simulink model "SmallScaleMicroGrid"  (R2023b)
settings: Solver=ode23tb  StartTime=0.0  StopTime=24*60*60  FixedStep=1/(1000)  MaxStep=60  RelTol=1e-4
PreLoadFcn:
  | load('SmallScaleMicroGridSolarLoadData24h.mat')
undefined symbols (not defined in the file): Angle, HPD_1min, HPT_1min, Magnitude, SPD_1min, SPT_1min
libraries: spsCurrentMeasurementLib x7, spsControlledCurrentSourceLib x5, spsSeriesRLCBranchLib x5, simulink x4, spsSeriesRLCLoadLib x3, spsVoltageMeasurementLib x2, spsThreePhaseTransformerTwoWindingsLib x1, spsGroundLib x1, spsLinearTransformerLib x1, spsPowerPhasorLib x1, spsThreePhasePISectionLineLib x1, spsThreePhaseSourceLib x1
settings Model: ModifiedByFormat=SPS  Creator=The MathWorks, Inc.  LastModifiedBy=SPS
settings SolverCC: InitialStep=1e-4  ZeroCrossAlgorithm=Adaptive  AlgebraicLoopSolver=TrustRegion
settings DataIOCC: SaveFormat=Array  SaveOutput=off  SaveTime=off  ReturnWorkspaceOutputs=off  SignalLoggingName=sigsOut
settings OptimizationCC: BooleanDataType=off  ExpressionDepthLimit=2147483647  InitFltsAndDblsToZero=on  LifeSpan=inf
settings DebuggingCC: AlgebraicLoopMsg=none  SaveWithParameterizedLinksMsg=none  UnderspecifiedInitializationDetection=Classic  MergeDetectMultiDrivingBlocksExec=none  SignalResolutionControl=TryResolveAllWithWarning  MultiTaskDSMMsg=warning  MultiTaskCondExecSysMsg=none  FcnCallInpInsideContextMsg=warning  UnconnectedInputMsg=warning  UnconnectedOutputMsg=warning  UnconnectedLineMsg=warning  AllowSymbolicDim=off  StateNameClashWarn=warning  SubsystemReferenceDiagnosticForUnitTest=warning  SFUnexpectedBacktrackingDiag=warning  SFNoUnconditionalDefaultTransitionDiag=warning  SFExecutionAtInitializationDiag=none  ArithmeticOperatorsInVariantConditions=warning
settings HardwareCC: ProdBitPerPointer=32  ProdBitPerSizeT=32  ProdBitPerPtrDiffT=32  ProdLargestAtomicFloat=None  ProdIntDivRoundTo=Undefined  ProdEndianess=Unspecified  ProdWordSize=32  ProdHWDeviceType=32-bit Generic  TargetUnknown=on
settings ModelReferenceCC: EnableRefExpFcnMdlSchedulingChecks=on  PropagateSignalLabelsOutOfModel=off
settings SFSimCC: SimUseLocalCustomCode=off  CustomCodeUndefinedFunction=UseInterfaceOnly
settings RTWCC: RTWUseLocalCustomCode=off  DLArmComputeVersion=19.05
settings CodeAppCC: StateflowObjectComments=on
settings GRTTargetCC: TargetFcnLib=ansi_tfl_tmw.mat  TargetLangStandard=C89/C90 (ANSI)  CombineOutputUpdateFcns=off  GRTInterface=on
settings ConfigComp: CovMetricSettings=dw  CovSaveCumulativeToWorkspaceVar=on  CovSaveSingleToWorkspaceVar=on  CovExternalEMLEnable=off  CovSFcnEnable=off
settings SimscapeCC: SimscapeNormalizeSystem=off

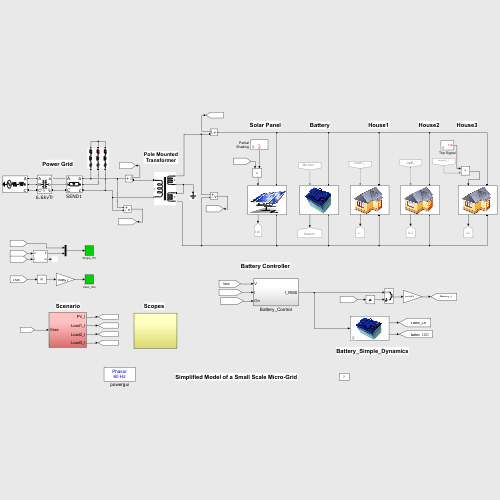
[thumbnail: Simulink's stored preview of the top-level diagram]
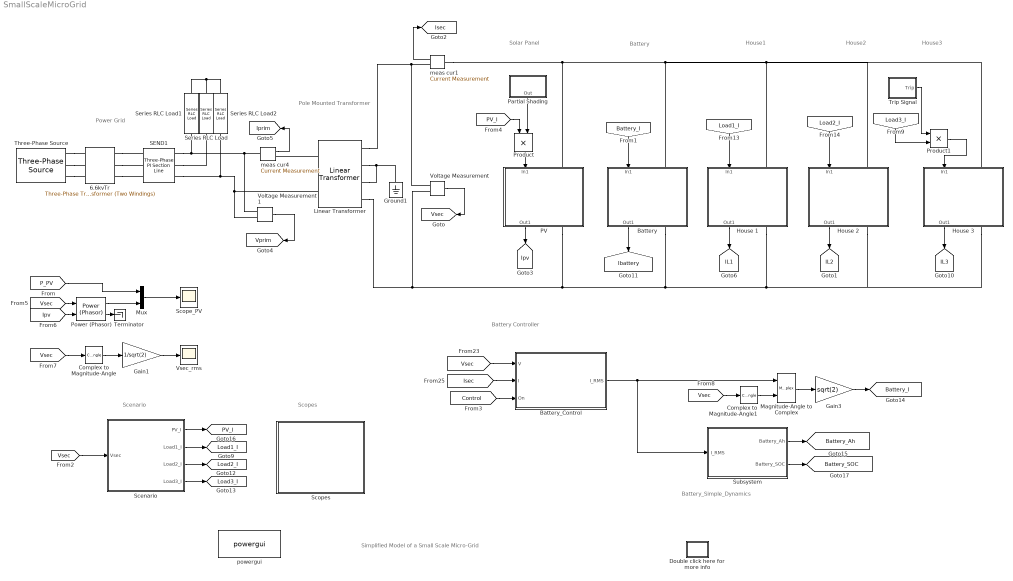
== system SmallScaleMicroGrid ==
  note: Power Grid
  note: Pole Mounted
      | Transformer
  note: Solar Panel
  note: Battery
  note: House1
  note: House2
  note: House3
  note: Battery_Simple_Dynamics
  note: Battery Controller
  note: Scenario
  note: Scopes
  note: Simplified Model of a Small Scale Micro-Grid
  6.6kvTr : spsThreePhaseTransformerTwoWindingsLib/Three-Phase Transformer (Two Windings)  Winding1Connection=Yg  Winding2Connection=Y  CoreType=Three single-phase transformers  SetSaturation=off  Hysteresis=off  DataFile='hysteresis'  SetInitialFlux=off  Measurements=None  UNITS=pu  NominalPower=[ 10e6 , 60 ]  Winding1=[ 66e3 , 0.002 , 0.08 ]  Winding2=[6.6e3 , 0.002 , 0.08 ]  Rm=500  Lm=500  L0=0.5  Saturation=[ 0,0 ; 0.0024,1.2 ; 1.0,1.52 ]  InitialFluxes=[ 0.8 , -0.8 , 0.7 ]  BreakLoop=on  DiscreteSolver=Trapezoidal iterative  DataType=off  TransfoNumber=1
  Battery : Subsystem
      mask Display: image('$imagefile')
  Battery_Control : Subsystem
  Complex to Magnitude-Angle : ComplexToMagnitudeAngle  Output=Magnitude
  Complex to Magnitude-Angle1 : ComplexToMagnitudeAngle  Output=Angle
  Double click here for more info : Subsystem
      settings: OpenFcn="showExample(\"simscapeelectricalsps/SmallScaleMicroGridExample\")"
      mask Display: disp('?')
  Gain1 : Gain  Gain=1/sqrt(2)
  Gain3 : Gain  Gain=sqrt(2)
  Ground1 : spsGroundLib/Ground  LConnTagsString=a
  House 1 : Subsystem
      mask Display: image('$imagefile')
  House 2 : Subsystem
      mask Display: image('$imagefile')
  House 3 : Subsystem
      mask Display: image('$imagefile')
  Linear Transformer : spsLinearTransformerLib/Linear Transformer  UNITS=pu  NominalPower=[75e3 60]  winding1=[ 6600 0.00005 0.0002 ]  winding2=[ 100 0.00005 0.0002 ]  ThreeWindings=on  winding3=[ 100 0.00005 0.0002 ]  RmLm=[ 50 50 ]  Measurements=None  DataType=off
  Magnitude-Angle to Complex : MagnitudeAngleToComplex
  Mux : Mux  Inputs=2
  PV : Subsystem
      mask Display: image('$imagefile')
  Partial Shading : Subsystem  mask(Signal Disturbance){Hour=11, Minute=0, Second=0, Duration=20, Factor=0.3}
      mask prompts: Duration "Duration (s):"
      mask help: Within the specified time range defined by Start and Duration parameters, output is set to 'Factor'. Outside the specified time range output is kept at 1.0.
      mask init:
      | T2=(Hour-1)*60*60;    % Hour in seconds
      | T3=(Minute-1)*60;  % Minute in seconds
      | Ton=T2+T3+(Second-1);    % Beginning of fault (s)
      | Toff=Ton+Duration; % End of fault (s)
      mask TypeOptions Hour: 0 |      1 |      2 |      3 |      4 |      5 |      6 |      7 |      8 |      9 |     10 |     11 |     12 |     13 |     14 |     15 |     16 |     17 |     18 |     19 |     20 |     21 |     22 |     23
      mask TypeOptions Minute: 0 |      1 |      2 |      3 |      4 |      5 |      6 |      7 |      8 |      9 |     10 |     11 |     12 |     13 |     14 |     15 |     16 |     17 |     18 |     19 |     20 |     21 |     22 |     23 |     24 |     25 |     26 |     27 |     28 |     29 |     30 |     31 |     32 |     33 |     34 |     35 |     36 |     37 |     38 |     39 |     40 |     41 |     42 |     43 |     44 |     45 |     46 |     47 |     48 |     49 |     50 |     51 |     52 |     53 |     54 |     55 |     56 |     57 |     58 |     59
      mask TypeOptions Second: 0 |      1 |      2 |      3 |      4 |      5 |      6 |      7 |      8 |      9 |     10 |     11 |     12 |     13 |     14 |     15 |     16 |     17 |     18 |     19 |     20 |     21 |     22 |     23 |     24 |     25 |     26 |     27 |     28 |     29 |     30 |     31 |     32 |     33 |     34 |     35 |     36 |     37 |     38 |     39 |     40 |     41 |     42 |     43 |     44 |     45 |     46 |     47 |     48 |     49 |     50 |     51 |     52 |     53 |     54 |     55 |     56 |     57 |     58 |     59
      mask DialogControl Control2 Prompt: Start:
  Power (Phasor) : spsPowerPhasorLib/Power (Phasor)
  Product : Product
  Product1 : Product
  SEND1 : spsThreePhasePISectionLineLib/Three-Phase PI Section Line  LConnTagsString=a|b|c  RConnTagsString=A|B|C  Length=1  Frequency=60  Resistances=[ 0.01273 0.3864]  Inductances="[ 0.9337e-3  4.1264e-3]"  Capacitances=[12.74e-9 7.751e-9]
  Scenario : Subsystem
  Scope_PV : Scope
  Scopes : Subsystem
  Series RLC Load : spsSeriesRLCLoadLib/Series RLC Load  LConnTagsString=a  RConnTagsString=__new0  NominalVoltage=1000  NominalFrequency=60  ActivePower=10e3  InductivePower=100  CapacitivePower=100  Setx0=off  InitialVoltage=0  SetiL0=off  InitialCurrent=0  Measurements=None  LoadType=constant Z
  Series RLC Load1 : spsSeriesRLCLoadLib/Series RLC Load  LConnTagsString=a  RConnTagsString=__new0  NominalVoltage=1000  NominalFrequency=60  ActivePower=100e3  InductivePower=100  CapacitivePower=100  Setx0=off  InitialVoltage=0  SetiL0=off  InitialCurrent=0  Measurements=None  LoadType=constant Z
  Series RLC Load2 : spsSeriesRLCLoadLib/Series RLC Load  LConnTagsString=a  RConnTagsString=__new0  NominalVoltage=1000  NominalFrequency=60  ActivePower=10e3  InductivePower=100  CapacitivePower=100  Setx0=off  InitialVoltage=0  SetiL0=off  InitialCurrent=0  Measurements=None  LoadType=constant Z
  Subsystem : Subsystem  mask{AH=1000}
      mask prompts: AH "Capacity[Ah]"
      mask Display: image('$imagefile')
  Terminator : Terminator
  Three-Phase Source : spsThreePhaseSourceLib/Three-Phase Source  InternalConnection=Yg  VoltagePhases=off  Voltage=66e3  PhaseAngle=0  Voltage_phases=[25e3 25e3 25e3]/sqrt(3)  PhaseAngles_phases=[0 -120 +120]  Frequency=60  NonIdealSource=on  SpecifyImpedance=on  Resistance=0.8929  Inductance=16.58e-3  ShortCircuitLevel=100e6  BaseVoltage=25e3  XRratio=7  BusType=swing  Pref=0  Qref=0  Prefabc=[10e3, 10e3, 10e3]  Qrefabc=[0, 0, 0]  Qmin=-inf  Qmax=inf
  Trip Signal : Subsystem  mask(Trip Signal for House Main Breaker){Hour=8, Minute=0, Second=0, FaultDuration=10}
      mask prompts: FaultDuration "Fault duration (s):"
      mask init:
      | T2=(Hour-1)*60*60;    % Hour in seconds
      | T3=(Minute-1)*60;  % Minute in seconds
      | Ton=T2+T3+(Second-1);    % Beginning of fault (s)
      | Toff=Ton+FaultDuration; % End of fault (s)
      mask TypeOptions Hour: 0 |      1 |      2 |      3 |      4 |      5 |      6 |      7 |      8 |      9 |     10 |     11 |     12 |     13 |     14 |     15 |     16 |     17 |     18 |     19 |     20 |     21 |     22 |     23
      mask TypeOptions Minute: 0 |      1 |      2 |      3 |      4 |      5 |      6 |      7 |      8 |      9 |     10 |     11 |     12 |     13 |     14 |     15 |     16 |     17 |     18 |     19 |     20 |     21 |     22 |     23 |     24 |     25 |     26 |     27 |     28 |     29 |     30 |     31 |     32 |     33 |     34 |     35 |     36 |     37 |     38 |     39 |     40 |     41 |     42 |     43 |     44 |     45 |     46 |     47 |     48 |     49 |     50 |     51 |     52 |     53 |     54 |     55 |     56 |     57 |     58 |     59
      mask TypeOptions Second: 0 |      1 |      2 |      3 |      4 |      5 |      6 |      7 |      8 |      9 |     10 |     11 |     12 |     13 |     14 |     15 |     16 |     17 |     18 |     19 |     20 |     21 |     22 |     23 |     24 |     25 |     26 |     27 |     28 |     29 |     30 |     31 |     32 |     33 |     34 |     35 |     36 |     37 |     38 |     39 |     40 |     41 |     42 |     43 |     44 |     45 |     46 |     47 |     48 |     49 |     50 |     51 |     52 |     53 |     54 |     55 |     56 |     57 |     58 |     59
      mask DialogControl Control2 Prompt: Fault timing:
  Voltage Measurement : spsVoltageMeasurementLib/Voltage Measurement  PhasorSimulation=on  OutputType=Complex  PSBequivalent=0
  Voltage Measurement1 : spsVoltageMeasurementLib/Voltage Measurement  PhasorSimulation=on  OutputType=Magnitude-Angle  PSBequivalent=0
  Vsec_rms : Scope
  meas cur1 : spsCurrentMeasurementLib/Current Measurement  PhasorSimulation=on  OutputType=Complex  PSBequivalent=0
  meas cur4 : spsCurrentMeasurementLib/Current Measurement  PhasorSimulation=on  OutputType=Magnitude-Angle  PSBequivalent=0
  powergui : spspowerguiLib/powergui  SimulationMode=Phasor  SampleTime=1/60/100  frequency=60  Iterations=50  frequencyindice=60  Pbase=100e6  ErrMax=1e-4  UnitsV=kV  UnitsW=MW  buscounter=0  FunctionMessages=off  echomessages=off  EnableUseOfTLC=off  CurrentSourceSwitches=off  DisableSnubberDevices=off  DisableRonSwitches=off  DisableVfSwitches=off  DisplayEquations=off  AutomaticDiscreteSolvers=off  SolverType=Tustin  Interpol=off  ExternalGateDelay=off  methode=off  Ts=0  x0status=blocks  SPID=off  SwTol=0  HookPort=off  NonlinearTolerance=0  nMaxIteration=15  ContinueOnMaxIteration=off  RestoreLinks=warning  ResistiveCurrentMeasurement=off  Frange=[0:2:500]  Ylog=off  Xlog=on  ShowGrid=off  save=off  variable=ZData  structure=0  ZoomFFT=on  StartTime=0.0  cycles=1  DisplayStyle=1  fundamental=60  FreqAxis=off  MaxFrequency=1000  frequencyindicesteady=1  RmsSteady=1  display=off
  tag scope: Battery_Ah=global, Battery_I=global, Battery_SOC=global, IL1=global, IL2=global, IL3=global, Ibattery=global, Iprim=global, Ipv=global, Isec=global, Load1_I=global, Load2_I=global, Load3_I=global, PV_I=global, Vprim=global, Vsec=global
  wires:
  House 2/1(Out1) -> [IL2]
  House 1/1(Out1) -> [IL1]
  meas cur1/1 -> [Isec]
  House 3/1(Out1) -> [IL3]
  [Load2_I] -> House 2/1(In1)
  Product1/1 -> House 3/1(In1)
  [Battery_I] -> Battery/1(In1)
  Subsystem/1(Battery_Ah) -> [Battery_Ah]
  Subsystem/2(Battery_SOC) -> [Battery_SOC]
  PV/1(Out1) -> [Ipv]
  Battery/1(Out1) -> [Ibattery]
  Scenario/1(PV_I) -> [PV_I]
  Scenario/2(Load1_I) -> [Load1_I]
  Scenario/3(Load2_I) -> [Load2_I]
  Scenario/4(Load3_I) -> [Load3_I]
  [Vsec] -> Scenario/1(Vsec)
  Voltage Measurement1/1 -> [Vprim]
  meas cur4/1 -> [Iprim]
  [Load1_I] -> House 1/1(In1)
  Voltage Measurement/1 -> [Vsec]
  [Isec] -> Battery_Control/2(I)
  [Vsec] -> Battery_Control/1(V)
  [Control] -> Battery_Control/3(On)
  [PV_I] -> Product/1
  Product/1 -> PV/1(In1)
  Partial Shading/1(Out) -> Product/2
  Mux/1 -> Scope_PV/1
  Power (Phasor)/1 -> Mux/2
  [Vsec] -> Power (Phasor)/1
  [Vsec] -> Complex to Magnitude-Angle/1
  Complex to Magnitude-Angle/1 -> Gain1/1
  [Ipv] -> Power (Phasor)/2
  Power (Phasor)/2 -> Terminator/1
  Gain1/1 -> Vsec_rms/1
  [P_PV] -> Mux/1
  Trip Signal/1(Trip) -> Product1/1
  [Load3_I] -> Product1/2
  Complex to Magnitude-Angle1/1 -> Magnitude-Angle to Complex/2
  Battery_Control/1(I_RMS) -> Subsystem/1(I_RMS), Magnitude-Angle to Complex/1
  Magnitude-Angle to Complex/1 -> Gain3/1
  [Vsec] -> Complex to Magnitude-Angle1/1
  Gain3/1 -> [Battery_I]
  connections:
  SEND1/RConn1 -- meas cur4/LConn1 -- Voltage Measurement1/LConn1 -- Series RLC Load1/RConn1
  SEND1/RConn3 -- Linear Transformer/LConn2 -- Voltage Measurement1/LConn2 -- Series RLC Load2/RConn1
  6.6kvTr/RConn2 -- SEND1/LConn2
  6.6kvTr/RConn1 -- SEND1/LConn1
  Three-Phase Source/RConn1 -- 6.6kvTr/LConn1
  Three-Phase Source/RConn3 -- 6.6kvTr/LConn3
  6.6kvTr/RConn3 -- SEND1/LConn3
  Ground1/LConn1 -- Linear Transformer/RConn3 -- Linear Transformer/RConn2
  Three-Phase Source/RConn2 -- 6.6kvTr/LConn2
  SEND1/RConn2 -- Series RLC Load/RConn1
  Series RLC Load1/LConn1 -- Series RLC Load/LConn1 -- Series RLC Load2/LConn1
  Linear Transformer/LConn1 -- meas cur4/RConn1
  Voltage Measurement/LConn1 -- meas cur1/RConn1 -- Linear Transformer/RConn1
  Voltage Measurement/LConn2 -- Battery/RConn1 -- House 1/RConn1 -- House 3/RConn1 -- House 2/RConn1 -- PV/RConn1 -- Linear Transformer/RConn4
  meas cur1/LConn1 -- PV/LConn1 -- Battery/LConn1 -- House 1/LConn1 -- House 2/LConn1 -- House 3/LConn1

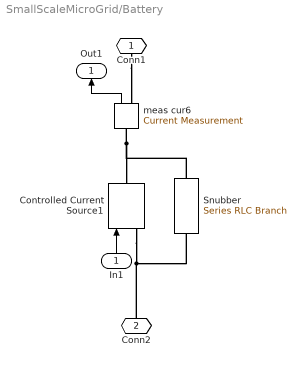
== system SmallScaleMicroGrid/Battery ==
  In1 : Inport
  Controlled Current Source1 : spsControlledCurrentSourceLib/Controlled Current Source  Initialize=on  Source_Type=AC  Amplitude=0  Phase=30  Frequency=60  Measurements=None
  Snubber : spsSeriesRLCBranchLib/Series RLC Branch  LConnTagsString=__new0  RConnTagsString=__new0  BranchType=R  Resistance=1e6  Inductance=1e-3  SetiL0=off  InitialCurrent=0  Capacitance=1e-6  Setx0=off  InitialVoltage=0  Measurements=None
  meas cur6 : spsCurrentMeasurementLib/Current Measurement  PhasorSimulation=on  OutputType=Complex  PSBequivalent=0
  Conn1 : PMIOPort  Side=Left
  Conn2 : PMIOPort  Port=2  Side=Right
  Out1 : Outport  VectorParamsAs1DForOutWhenUnconnected=off
  wires:
  meas cur6/1 -> Out1/1
  In1/1 -> Controlled Current Source1/1
  connections:
  Conn2/RConn1 -- Controlled Current Source1/LConn1 -- Snubber/RConn1
  meas cur6/LConn1 -- Controlled Current Source1/RConn1 -- Snubber/LConn1
  Conn1/RConn1 -- meas cur6/RConn1

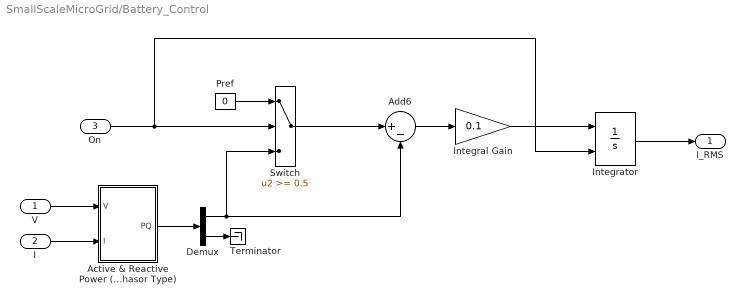
== system SmallScaleMicroGrid/Battery_Control ==
  V : Inport
  I : Inport  Port=2
  On : Inport  Port=3
  Active & Reactive Power (Phasor Type) : Subsystem  DialogController=POWERSYS.PowerSysDialog  mask(Active & Reactive Power (Phasor Type)){}
      mask help: Active & Reactive Power (Phasor Type)
      mask init:
      | power_initmask();
      mask Help: This block is part of a subset of blocks in the Extras library that does not have documentation associated with it, other than the block mask description.
      mask Display: disp('')
  Add6 : Sum  Inputs=|+-
  Demux : Demux  Outputs=2
  Integral Gain : Gain  Gain=0.1
  Integrator : Integrator  ExternalReset=falling  LimitOutput=on  UpperSaturationLimit=50  LowerSaturationLimit=-50
  Pref : Constant  Value=0
  Switch : Switch  Threshold=0.5  SaturateOnIntegerOverflow=off  InputSameDT=off
  Terminator : Terminator
  I_RMS : Outport  OutputWhenDisabled=reset  InitialOutput=0  VectorParamsAs1DForOutWhenUnconnected=off
  wires:
  Pref/1 -> Switch/1
  Integrator/1 -> I_RMS/1
  On/1 -> Integrator/2, Switch/2
  Add6/1 -> Integral Gain/1
  Integral Gain/1 -> Integrator/1
  Demux/1 -> Switch/3, Add6/2
  Active & Reactive Power (Phasor Type)/1(PQ) -> Demux/1
  I/1 -> Active & Reactive Power (Phasor Type)/2(I)
  V/1 -> Active & Reactive Power (Phasor Type)/1(V)
  Demux/2 -> Terminator/1
  Switch/1 -> Add6/1

== system SmallScaleMicroGrid/Double click here for more info ==

== system SmallScaleMicroGrid/House 1 ==
  In1 : Inport
  Controlled Current Source4 : spsControlledCurrentSourceLib/Controlled Current Source  Initialize=on  Source_Type=AC  Amplitude=0  Phase=30  Frequency=60  Measurements=None
  Snubber3 : spsSeriesRLCBranchLib/Series RLC Branch  LConnTagsString=__new0  RConnTagsString=__new0  BranchType=R  Resistance=1e6  Inductance=1e-3  SetiL0=off  InitialCurrent=0  Capacitance=1e-6  Setx0=off  InitialVoltage=0  Measurements=None
  meas cur2 : spsCurrentMeasurementLib/Current Measurement  PhasorSimulation=on  OutputType=Complex  PSBequivalent=0
  Conn1 : PMIOPort  Side=Left
  Conn2 : PMIOPort  Port=2  Side=Right
  Out1 : Outport  VectorParamsAs1DForOutWhenUnconnected=off
  wires:
  meas cur2/1 -> Out1/1
  In1/1 -> Controlled Current Source4/1
  connections:
  Controlled Current Source4/LConn1 -- Conn2/RConn1 -- Snubber3/RConn1
  Controlled Current Source4/RConn1 -- Snubber3/LConn1 -- meas cur2/RConn1
  meas cur2/LConn1 -- Conn1/RConn1

== system SmallScaleMicroGrid/House 2 ==
  In1 : Inport
  Controlled Current Source4 : spsControlledCurrentSourceLib/Controlled Current Source  Initialize=on  Source_Type=AC  Amplitude=0  Phase=30  Frequency=60  Measurements=None
  Snubber3 : spsSeriesRLCBranchLib/Series RLC Branch  LConnTagsString=__new0  RConnTagsString=__new0  BranchType=R  Resistance=1e6  Inductance=1e-3  SetiL0=off  InitialCurrent=0  Capacitance=1e-6  Setx0=off  InitialVoltage=0  Measurements=None
  meas cur2 : spsCurrentMeasurementLib/Current Measurement  PhasorSimulation=on  OutputType=Complex  PSBequivalent=0
  Conn1 : PMIOPort  Side=Left
  Conn2 : PMIOPort  Port=2  Side=Right
  Out1 : Outport  VectorParamsAs1DForOutWhenUnconnected=off
  wires:
  meas cur2/1 -> Out1/1
  In1/1 -> Controlled Current Source4/1
  connections:
  Snubber3/LConn1 -- Controlled Current Source4/RConn1 -- meas cur2/RConn1
  Conn2/RConn1 -- Controlled Current Source4/LConn1 -- Snubber3/RConn1
  Conn1/RConn1 -- meas cur2/LConn1

== system SmallScaleMicroGrid/House 3 ==
  In1 : Inport
  Controlled Current Source4 : spsControlledCurrentSourceLib/Controlled Current Source  Initialize=on  Source_Type=AC  Amplitude=0  Phase=30  Frequency=60  Measurements=None
  Snubber3 : spsSeriesRLCBranchLib/Series RLC Branch  LConnTagsString=__new0  RConnTagsString=__new0  BranchType=R  Resistance=1e6  Inductance=1e-3  SetiL0=off  InitialCurrent=0  Capacitance=1e-6  Setx0=off  InitialVoltage=0  Measurements=None
  meas cur2 : spsCurrentMeasurementLib/Current Measurement  PhasorSimulation=on  OutputType=Complex  PSBequivalent=0
  Conn1 : PMIOPort  Side=Left
  Conn2 : PMIOPort  Port=2  Side=Right
  Out1 : Outport  VectorParamsAs1DForOutWhenUnconnected=off
  wires:
  meas cur2/1 -> Out1/1
  In1/1 -> Controlled Current Source4/1
  connections:
  Controlled Current Source4/RConn1 -- Snubber3/LConn1 -- meas cur2/RConn1
  Controlled Current Source4/LConn1 -- Conn2/RConn1 -- Snubber3/RConn1
  meas cur2/LConn1 -- Conn1/RConn1

== system SmallScaleMicroGrid/PV ==
  In1 : Inport
  Controlled Current Source : spsControlledCurrentSourceLib/Controlled Current Source  Initialize=on  Source_Type=AC  Amplitude=0  Phase=30  Frequency=60  Measurements=None
  Snubber1 : spsSeriesRLCBranchLib/Series RLC Branch  LConnTagsString=__new0  RConnTagsString=__new0  BranchType=R  Resistance=1e6  Inductance=1e-3  SetiL0=off  InitialCurrent=0  Capacitance=1e-6  Setx0=off  InitialVoltage=0  Measurements=None
  meas cur3 : spsCurrentMeasurementLib/Current Measurement  PhasorSimulation=on  OutputType=Complex  PSBequivalent=0
  Conn1 : PMIOPort  Side=Left
  Conn2 : PMIOPort  Port=2  Side=Right
  Out1 : Outport  VectorParamsAs1DForOutWhenUnconnected=off
  wires:
  In1/1 -> Controlled Current Source/1
  meas cur3/1 -> Out1/1
  connections:
  meas cur3/LConn1 -- Snubber1/LConn1 -- Controlled Current Source/RConn1
  Snubber1/RConn1 -- Controlled Current Source/LConn1 -- Conn2/RConn1
  Conn1/RConn1 -- meas cur3/RConn1

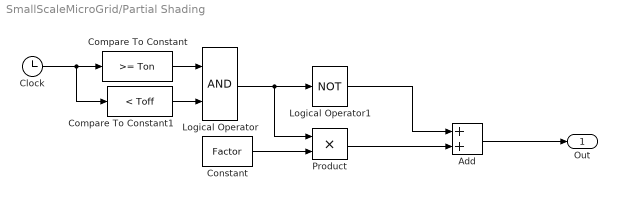
== system SmallScaleMicroGrid/Partial Shading ==
  Add : Sum
  Clock : Clock
  Compare To Constant : simulink/Logic and Bit Operations/Compare To Constant  relop=>=  const=Ton  OutDataTypeStr=boolean
  Compare To Constant1 : simulink/Logic and Bit Operations/Compare To Constant  relop=<  const=Toff  OutDataTypeStr=boolean
  Constant : Constant  Value=Factor
  Logical Operator : Logic  AllPortsSameDT=off  OutDataTypeStr=float('double')
  Logical Operator1 : Logic  Operator=NOT  AllPortsSameDT=off  OutDataTypeStr=float('double')
  Product : Product
  Out : Outport  VectorParamsAs1DForOutWhenUnconnected=off
  wires:
  Add/1 -> Out/1
  Product/1 -> Add/2
  Constant/1 -> Product/2
  Compare To Constant/1 -> Logical Operator/1
  Clock/1 -> Compare To Constant1/1, Compare To Constant/1
  Compare To Constant1/1 -> Logical Operator/2
  Logical Operator/1 -> Logical Operator1/1, Product/1
  Logical Operator1/1 -> Add/1

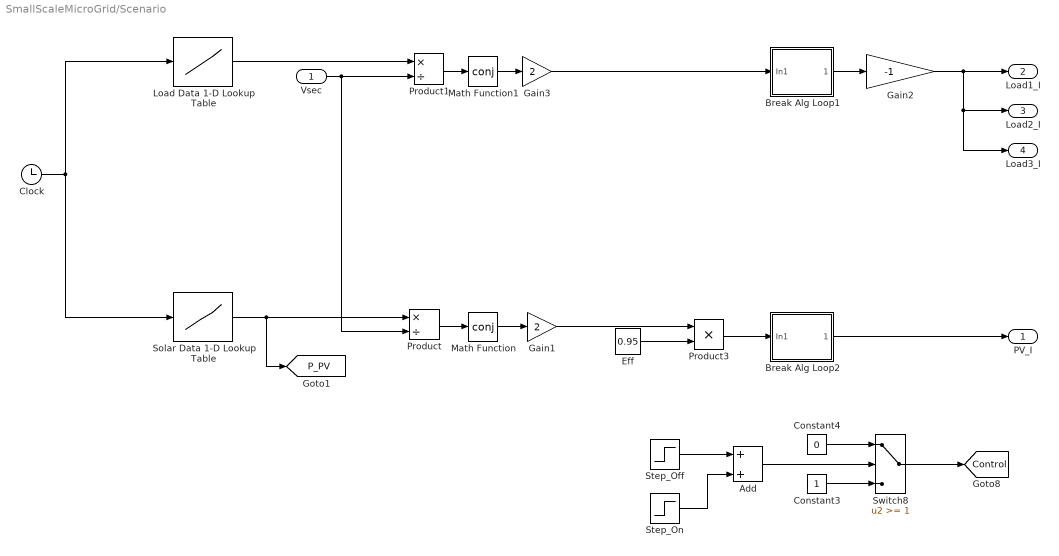
== system SmallScaleMicroGrid/Scenario ==
  Vsec : Inport
  Add : Sum
  Break Alg Loop1 : Subsystem
  Break Alg Loop2 : Subsystem
  Clock : Clock
  Constant3 : Constant
  Constant4 : Constant  Value=0
  Eff : Constant  Value=0.95
  Gain1 : Gain  Gain=2
  Gain2 : Gain  Gain=-1
  Gain3 : Gain  Gain=2
  Load Data 1-D Lookup Table : Lookup_n-D  NumberOfTableDimensions=1  BreakpointsForDimension1=HPT_1min  BeginIndexSearchUsingPreviousIndexResult=on  Table=HPD_1min  InternalRulePriority=Speed  RndMeth=Simplest
  Math Function : Math  Operator=conj
  Math Function1 : Math  Operator=conj
  Product : Product  Inputs=*/
  Product1 : Product  Inputs=*/
  Product3 : Product  Inputs=**
  Solar Data 1-D Lookup Table : Lookup_n-D  NumberOfTableDimensions=1  BreakpointsForDimension1=SPT_1min  BeginIndexSearchUsingPreviousIndexResult=on  Table=SPD_1min  InternalRulePriority=Speed  RndMeth=Simplest
  Step_Off : Step  Time=12*60*60  SampleTime=0
  Step_On : Step  Time=18*60*60  After=-1  SampleTime=0
  Switch8 : Switch  Threshold=1  SaturateOnIntegerOverflow=off  InputSameDT=off
  PV_I : Outport  VectorParamsAs1DForOutWhenUnconnected=off
  Load1_I : Outport  Port=2  VectorParamsAs1DForOutWhenUnconnected=off
  Load2_I : Outport  Port=3  VectorParamsAs1DForOutWhenUnconnected=off
  Load3_I : Outport  Port=4  VectorParamsAs1DForOutWhenUnconnected=off
  tag scope: Control=global, P_PV=global
  wires:
  Step_On/1 -> Add/2
  Eff/1 -> Product3/2
  Break Alg Loop1/1("1 ") -> Gain2/1
  Math Function/1 -> Gain1/1
  Product3/1 -> Break Alg Loop2/1(In1)
  Gain3/1 -> Break Alg Loop1/1(In1)
  Clock/1 -> Solar Data 1-D Lookup Table/1, Load Data 1-D Lookup Table/1
  Gain1/1 -> Product3/1
  Add/1 -> Switch8/2
  Math Function1/1 -> Gain3/1
  Solar Data 1-D Lookup Table/1 -> Product/1, [P_PV]
  Constant4/1 -> Switch8/1
  Break Alg Loop2/1("1 ") -> PV_I/1
  Product/1 -> Math Function/1
  Product1/1 -> Math Function1/1
  Load Data 1-D Lookup Table/1 -> Product1/1
  Gain2/1 -> Load3_I/1, Load2_I/1, Load1_I/1
  Switch8/1 -> [Control]
  Vsec/1 -> Product/2, Product1/2
  Step_Off/1 -> Add/1
  Constant3/1 -> Switch8/3

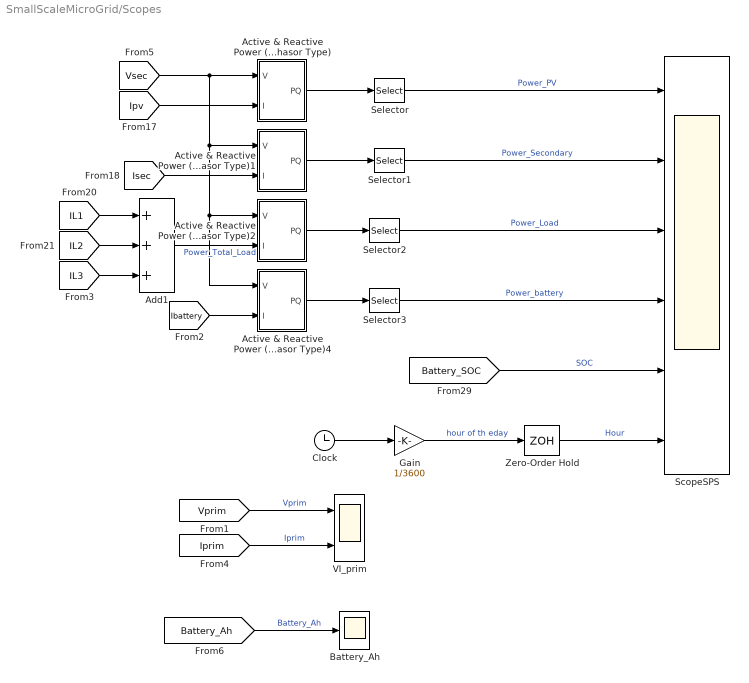
== system SmallScaleMicroGrid/Scopes ==
  Active & Reactive Power (Phasor Type) : Subsystem  DialogController=POWERSYS.PowerSysDialog  mask(Active & Reactive Power (Phasor Type)){}
      mask help: Active & Reactive Power (Phasor Type)
      mask init:
      | power_initmask();
      mask Help: This block is part of a subset of blocks in the Extras library that does not have documentation associated with it, other than the block mask description.
      mask Display: disp('')
  Active & Reactive Power (Phasor Type)1 : Subsystem  DialogController=POWERSYS.PowerSysDialog  mask(Active & Reactive Power (Phasor Type)){}
      mask help: Active & Reactive Power (Phasor Type)
      mask init:
      | power_initmask();
      mask Help: This block is part of a subset of blocks in the Extras library that does not have documentation associated with it, other than the block mask description.
      mask Display: disp('')
  Active & Reactive Power (Phasor Type)2 : Subsystem  DialogController=POWERSYS.PowerSysDialog  mask(Active & Reactive Power (Phasor Type)){}
      mask help: Active & Reactive Power (Phasor Type)
      mask init:
      | power_initmask();
      mask Help: This block is part of a subset of blocks in the Extras library that does not have documentation associated with it, other than the block mask description.
      mask Display: disp('')
  Active & Reactive Power (Phasor Type)4 : Subsystem  DialogController=POWERSYS.PowerSysDialog  mask(Active & Reactive Power (Phasor Type)){}
      mask help: Active & Reactive Power (Phasor Type)
      mask init:
      | power_initmask();
      mask Help: This block is part of a subset of blocks in the Extras library that does not have documentation associated with it, other than the block mask description.
      mask Display: disp('')
  Add1 : Sum  Inputs=+++
  Battery_Ah : Scope
  Clock : Clock
  Gain : Gain  Gain=1/3600
  ScopeSPS : Scope  NumInputPorts=6
  Selector{,1..3} (4 alike) : Selector  InputPortWidth=2  IndexOptions=Index vector (dialog)  Indices=1  OutputSizes=1
  VI_prim : Scope  NumInputPorts=2
  Zero-Order Hold : ZeroOrderHold  SampleTime=3600
  wires:
  [Ipv] -> Active & Reactive Power (Phasor Type)/2(I)
  [Vsec] -> Active & Reactive Power (Phasor Type)4/1(V), Active & Reactive Power (Phasor Type)2/1(V), Active & Reactive Power (Phasor Type)1/1(V), Active & Reactive Power (Phasor Type)/1(V)
  Active & Reactive Power (Phasor Type)/1(PQ) -> Selector/1
  Selector/1 -> ScopeSPS/1  "Power_PV"
  [IL1] -> Add1/1
  [IL2] -> Add1/2
  [IL3] -> Add1/3
  [Isec] -> Active & Reactive Power (Phasor Type)1/2(I)
  Add1/1 -> Active & Reactive Power (Phasor Type)2/2(I)  "Power_Total_Load"
  [Ibattery] -> Active & Reactive Power (Phasor Type)4/2(I)
  Active & Reactive Power (Phasor Type)1/1(PQ) -> Selector1/1
  Active & Reactive Power (Phasor Type)2/1(PQ) -> Selector2/1
  Active & Reactive Power (Phasor Type)4/1(PQ) -> Selector3/1
  Selector1/1 -> ScopeSPS/2  "Power_Secondary"
  Selector2/1 -> ScopeSPS/3  "Power_Load"
  Selector3/1 -> ScopeSPS/4  "Power_battery"
  [Battery_SOC] -> ScopeSPS/5  "SOC"
  [Vprim] -> VI_prim/1  "Vprim"
  [Iprim] -> VI_prim/2  "Iprim"
  [Battery_Ah] -> Battery_Ah/1  "Battery_Ah"
  Clock/1 -> Gain/1
  Gain/1 -> Zero-Order Hold/1  "hour of th eday"
  Zero-Order Hold/1 -> ScopeSPS/6  "Hour"

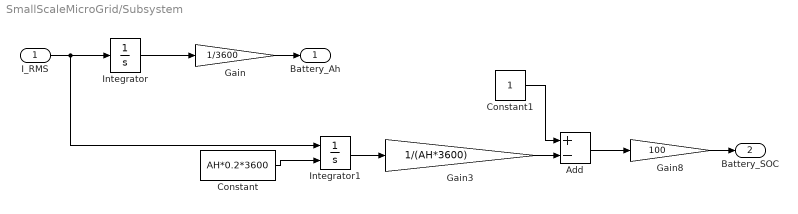
== system SmallScaleMicroGrid/Subsystem ==
  I_RMS : Inport
  Add : Sum  Inputs=+-
  Constant : Constant  Value=AH*0.2*3600
  Constant1 : Constant
  Gain : Gain  Gain=1/3600
  Gain3 : Gain  Gain=1/(AH*3600)
  Gain8 : Gain  Gain=100
  Integrator : Integrator
  Integrator1 : Integrator  InitialConditionSource=external
  Battery_Ah : Outport  VectorParamsAs1DForOutWhenUnconnected=off
  Battery_SOC : Outport  Port=2  VectorParamsAs1DForOutWhenUnconnected=off
  wires:
  Integrator/1 -> Gain/1
  Integrator1/1 -> Gain3/1
  Gain3/1 -> Add/2
  Constant1/1 -> Add/1
  Add/1 -> Gain8/1
  Constant/1 -> Integrator1/2
  I_RMS/1 -> Integrator/1, Integrator1/1
  Gain/1 -> Battery_Ah/1
  Gain8/1 -> Battery_SOC/1

== system SmallScaleMicroGrid/Trip Signal ==
  note: 0 = TRIP
  Clock : Clock
  Compare To Constant : simulink/Logic and Bit Operations/Compare To Constant  relop=>=  const=Ton  OutDataTypeStr=boolean
  Compare To Constant1 : simulink/Logic and Bit Operations/Compare To Constant  relop=<  const=Toff  OutDataTypeStr=boolean
  Logical Operator : Logic  AllPortsSameDT=off  OutDataTypeStr=float('double')
  Logical Operator1 : Logic  Operator=NOT  AllPortsSameDT=off  OutDataTypeStr=float('double')
  Trip : Outport  VectorParamsAs1DForOutWhenUnconnected=off
  wires:
  Compare To Constant/1 -> Logical Operator/1
  Clock/1 -> Compare To Constant1/1, Compare To Constant/1
  Compare To Constant1/1 -> Logical Operator/2
  Logical Operator/1 -> Logical Operator1/1
  Logical Operator1/1 -> Trip/1

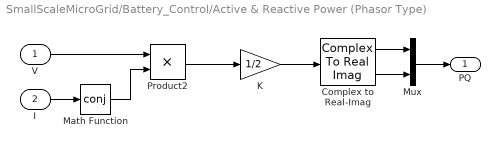
== system SmallScaleMicroGrid/Battery_Control/Active & Reactive Power (Phasor Type) ==
  V : Inport
  I : Inport  Port=2
  Complex to Real-Imag : ComplexToRealImag
  K : Gain  Gain=1/2  SaturateOnIntegerOverflow=on  OutDataTypeStr=Inherit: Same as input  ParamDataTypeStr=Inherit: Same as input
  Math Function : Math  Operator=conj  SignedPower=on
  Mux : Mux  Inputs=2
  Product2 : Product  InputSameDT=on  SaturateOnIntegerOverflow=on  OutDataTypeStr=Inherit: Same as first input
  PQ : Outport  VectorParamsAs1DForOutWhenUnconnected=off
  wires:
  Mux/1 -> PQ/1
  Complex to Real-Imag/2 -> Mux/2
  Complex to Real-Imag/1 -> Mux/1
  V/1 -> Product2/1
  Math Function/1 -> Product2/2
  Product2/1 -> K/1
  K/1 -> Complex to Real-Imag/1
  I/1 -> Math Function/1

== system SmallScaleMicroGrid/Scenario/Break Alg Loop1 ==
  In1 : Inport
  Complex to Real-Imag : ComplexToRealImag
  Real-Imag to Complex : RealImagToComplex
  Transfer Fcn : TransferFcn  Denominator=[1e-6 1]
  Transfer Fcn1 : TransferFcn  Denominator=[1e-6 1]
  "1 " : Outport
  wires:
  Transfer Fcn1/1 -> Real-Imag to Complex/2
  Real-Imag to Complex/1 -> "1 "/1
  Transfer Fcn/1 -> Real-Imag to Complex/1
  Complex to Real-Imag/2 -> Transfer Fcn1/1
  Complex to Real-Imag/1 -> Transfer Fcn/1
  In1/1 -> Complex to Real-Imag/1

== system SmallScaleMicroGrid/Scenario/Break Alg Loop2 ==
  In1 : Inport
  Complex to Real-Imag : ComplexToRealImag
  Real-Imag to Complex : RealImagToComplex
  Transfer Fcn : TransferFcn  Denominator=[1e-6 1]
  Transfer Fcn1 : TransferFcn  Denominator=[1e-6 1]
  "1 " : Outport
  wires:
  In1/1 -> Complex to Real-Imag/1
  Complex to Real-Imag/1 -> Transfer Fcn/1
  Complex to Real-Imag/2 -> Transfer Fcn1/1
  Transfer Fcn/1 -> Real-Imag to Complex/1
  Real-Imag to Complex/1 -> "1 "/1
  Transfer Fcn1/1 -> Real-Imag to Complex/2

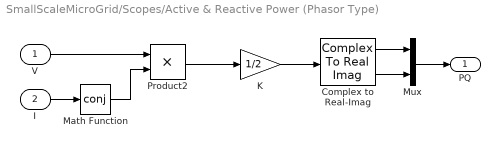
== system SmallScaleMicroGrid/Scopes/Active & Reactive Power (Phasor Type) ==
  V : Inport
  I : Inport  Port=2
  Complex to Real-Imag : ComplexToRealImag
  K : Gain  Gain=1/2  SaturateOnIntegerOverflow=on  OutDataTypeStr=Inherit: Same as input  ParamDataTypeStr=Inherit: Same as input
  Math Function : Math  Operator=conj  SignedPower=on
  Mux : Mux  Inputs=2
  Product2 : Product  InputSameDT=on  SaturateOnIntegerOverflow=on  OutDataTypeStr=Inherit: Same as first input
  PQ : Outport  VectorParamsAs1DForOutWhenUnconnected=off
  wires:
  Mux/1 -> PQ/1
  Complex to Real-Imag/2 -> Mux/2
  Complex to Real-Imag/1 -> Mux/1
  V/1 -> Product2/1
  Math Function/1 -> Product2/2
  Product2/1 -> K/1
  K/1 -> Complex to Real-Imag/1
  I/1 -> Math Function/1

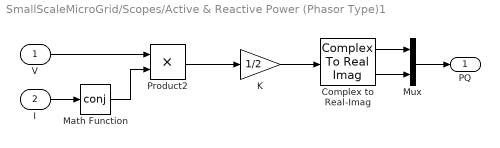
== system SmallScaleMicroGrid/Scopes/Active & Reactive Power (Phasor Type)1 ==
  V : Inport
  I : Inport  Port=2
  Complex to Real-Imag : ComplexToRealImag
  K : Gain  Gain=1/2  SaturateOnIntegerOverflow=on  OutDataTypeStr=Inherit: Same as input  ParamDataTypeStr=Inherit: Same as input
  Math Function : Math  Operator=conj  SignedPower=on
  Mux : Mux  Inputs=2
  Product2 : Product  InputSameDT=on  SaturateOnIntegerOverflow=on  OutDataTypeStr=Inherit: Same as first input
  PQ : Outport  VectorParamsAs1DForOutWhenUnconnected=off
  wires:
  Mux/1 -> PQ/1
  Complex to Real-Imag/2 -> Mux/2
  Complex to Real-Imag/1 -> Mux/1
  V/1 -> Product2/1
  Math Function/1 -> Product2/2
  Product2/1 -> K/1
  K/1 -> Complex to Real-Imag/1
  I/1 -> Math Function/1

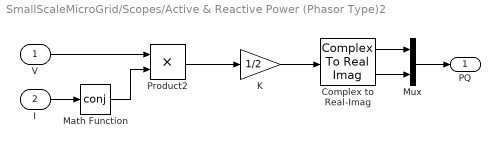
== system SmallScaleMicroGrid/Scopes/Active & Reactive Power (Phasor Type)2 ==
  V : Inport
  I : Inport  Port=2
  Complex to Real-Imag : ComplexToRealImag
  K : Gain  Gain=1/2  SaturateOnIntegerOverflow=on  OutDataTypeStr=Inherit: Same as input  ParamDataTypeStr=Inherit: Same as input
  Math Function : Math  Operator=conj  SignedPower=on
  Mux : Mux  Inputs=2
  Product2 : Product  InputSameDT=on  SaturateOnIntegerOverflow=on  OutDataTypeStr=Inherit: Same as first input
  PQ : Outport  VectorParamsAs1DForOutWhenUnconnected=off
  wires:
  Mux/1 -> PQ/1
  Complex to Real-Imag/2 -> Mux/2
  Complex to Real-Imag/1 -> Mux/1
  V/1 -> Product2/1
  Math Function/1 -> Product2/2
  Product2/1 -> K/1
  K/1 -> Complex to Real-Imag/1
  I/1 -> Math Function/1

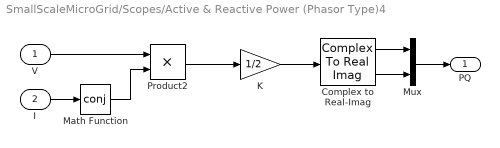
== system SmallScaleMicroGrid/Scopes/Active & Reactive Power (Phasor Type)4 ==
  V : Inport
  I : Inport  Port=2
  Complex to Real-Imag : ComplexToRealImag
  K : Gain  Gain=1/2  SaturateOnIntegerOverflow=on  OutDataTypeStr=Inherit: Same as input  ParamDataTypeStr=Inherit: Same as input
  Math Function : Math  Operator=conj  SignedPower=on
  Mux : Mux  Inputs=2
  Product2 : Product  InputSameDT=on  SaturateOnIntegerOverflow=on  OutDataTypeStr=Inherit: Same as first input
  PQ : Outport  VectorParamsAs1DForOutWhenUnconnected=off
  wires:
  Mux/1 -> PQ/1
  Complex to Real-Imag/2 -> Mux/2
  Complex to Real-Imag/1 -> Mux/1
  V/1 -> Product2/1
  Math Function/1 -> Product2/2
  Product2/1 -> K/1
  K/1 -> Complex to Real-Imag/1
  I/1 -> Math Function/1
